simulink model "Modified_MIT_model_Ster_Adaptacyjne_am_2017b"  (R2021b)
settings: Solver=FixedStepAuto  StartTime=0.0  StopTime=100  FixedStep=0.001  RelTol=1e-3
values from neighbouring files (symbols this model uses):
  alpha = 1    [Modified_MIT_skrypt_Ster_Adaptacyjne_am.m]
  gamma = gamma_vec(i)    [Modified_MIT_skrypt_Ster_Adaptacyjne_am.m]    (also in skrypt_Ster_Adaptacyjne.m; skrypt_Ster_Adaptacyjne_2_rzedu.m; skrypt_Ster_Adaptacyjne_am.m)
  kd = 0.01    [Modified_MIT_skrypt_Ster_Adaptacyjne_am.m]
  ki = 1    [Modified_MIT_skrypt_Ster_Adaptacyjne_am.m]
  kp = 5    [Modified_MIT_skrypt_Ster_Adaptacyjne_am.m]
libraries: slpidlib x2
settings Model: Creator=marci  LastModifiedBy=marci
settings DebuggingCC: UnconnectedInputMsg=none  UnconnectedOutputMsg=none  UnconnectedLineMsg=none
settings RTWCC: DLArmComputeVersion=20.02.1

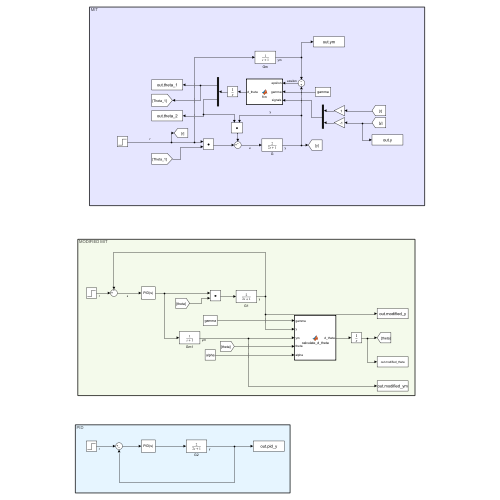
[thumbnail: Simulink's stored preview of the top-level diagram]
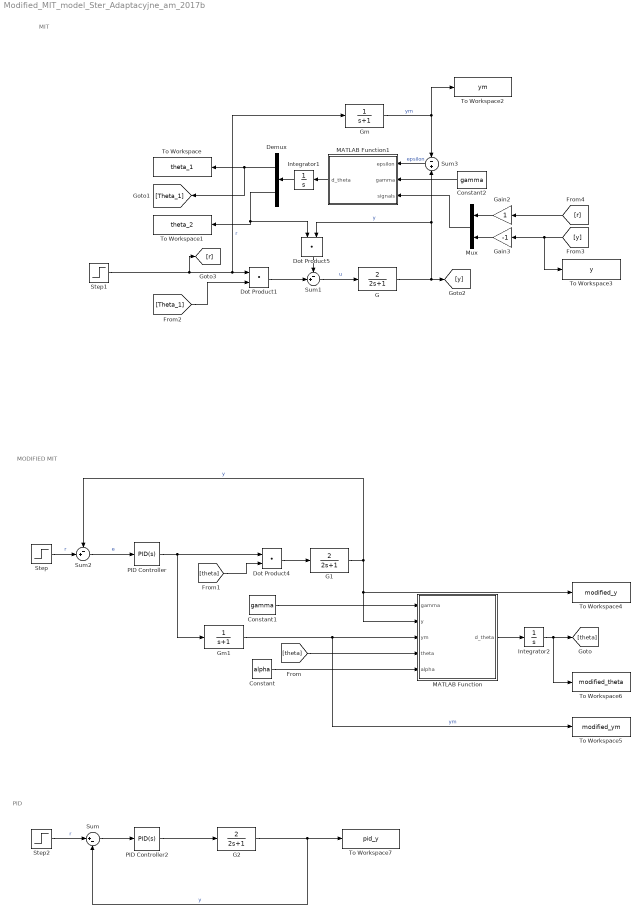
== system Modified_MIT_model_Ster_Adaptacyjne_am_2017b ==
  note: PID
  note: MODIFIED MIT
  note: MIT
  Constant : Constant  Value=alpha
  Constant1 : Constant  Value=gamma
  Constant2 : Constant  Value=gamma
  Demux : Demux  Outputs=2
  Dot Product1 : DotProduct  InputSameDT=on  OutDataTypeStr=Inherit: Inherit via internal rule
  Dot Product4 : DotProduct  InputSameDT=on  OutDataTypeStr=Inherit: Inherit via internal rule
  Dot Product5 : DotProduct  InputSameDT=on  OutDataTypeStr=Inherit: Inherit via internal rule
  G : TransferFcn  Numerator=[2]  Denominator=[2 1]
  G1 : TransferFcn  Numerator=[2]  Denominator=[2 1]
  G2 : TransferFcn  Numerator=[2]  Denominator=[2 1]
  Gain2 : Gain
  Gain3 : Gain  Gain=-1
  Gm : TransferFcn  Denominator=[1 1]
  Gm1 : TransferFcn  Denominator=[1 1]
  Integrator1 : Integrator
  Integrator2 : Integrator  InitialCondition=0.00001
  MATLAB Function : MATLAB Function  TreatAsAtomicUnit=on
  MATLAB Function1 : MATLAB Function  TreatAsAtomicUnit=on
  Mux : Mux  Inputs=2
  PID Controller : slpidlib/PID Controller  Controller=PID  Form=Parallel  TimeDomain=Continuous-time  UseExternalTs=off  SampleTime=-1  IntegratorMethod=Forward Euler  FilterMethod=Forward Euler  ControllerParametersSource=internal  P=kp  I=ki  D=kd  N=100  UseFilter=on  TunerSelectOption=Transfer Function Based (PID Tuner App)  InitialConditionSource=internal  InitialConditionForIntegrator=0  InitialConditionForFilter=0  DifferentiatorICPrevScaledInput=0  ExternalReset=none  TrackingMode=off  Kt=1  LimitOutput=off  SatLimitsSource=internal  UpperSaturationLimit=inf  LowerSaturationLimit=-inf  LinearizeAsGain=on  AntiWindupMode=none  Kb=1  POutMin=[]  POutMax=[]  IOutMin=[]  IOutMax=[]  DOutMin=[]  DOutMax=[]  NOutMin=[]  NOutMax=[]  SumOutMin=[]  SumOutMax=[]  SaturationOutMin=[]  SaturationOutMax=[]  PParamMin=[]  PParamMax=[]  IParamMin=[]  IParamMax=[]  DParamMin=[]  DParamMax=[]  NParamMin=[]  NParamMax=[]  KbParamMin=[]  KbParamMax=[]  KtParamMin=[]  KtParamMax=[]  KbOutMin=[]  KbOutMax=[]  KtOutMin=[]  KtOutMax=[]  IntegratorOutMin=[]  IntegratorOutMax=[]  FilterOutMin=[]  FilterOutMax=[]  SumI1OutMin=[]  SumI1OutMax=[]  SumI2OutMin=[]  SumI2OutMax=[]  SumI3OutMin=[]  SumI3OutMax=[]  SumI4OutMin=[]  SumI4OutMax=[]  SumDOutMin=[]  SumDOutMax=[]  DifferentiatorOutMin=[]  DifferentiatorOutMax=[]  FilterDiffOutCoefMin=[]  FilterDiffOutCoefMax=[]  ReciprocalOutMin=[]  ReciprocalOutMax=[]  SumDenOutMin=[]  SumDenOutMax=[]  SumNumOutMin=[]  SumNumOutMax=[]  DivideOutMin=[]  DivideOutMax=[]  UdiffTsProdOutMin=[]  UdiffTsProdOutMax=[]  NTsProdOutMin=[]  NTsProdOutMax=[]  UintegralTsProdOutMin=[]  UintegralTsProdOutMax=[]  UngainTsProdOutMin=[]  UngainTsProdOutMax=[]  IntegratorContinuousStateAttributes=''  IntegratorStateMustResolveToSignalObject=off  IntegratorRTWStateStorageClass=Auto  FilterContinuousStateAttributes=''  FilterStateMustResolveToSignalObject=off  FilterRTWStateStorageClass=Auto  ParallelPVariant=InternalParameters  IdealPVariant=Disabled  IVariant=InternalParameters  DVariant=InternalParameters  IntegratorVariant=Continuous  SatVariant=Disabled  AWVariant=Passthrough  PCopyVariant=Disabled  TRVariant=Disabled  FdbkBlocksVariant=Forward  IdealPFdbkVariant=Disabled  SatFdbkVariant=Disabled  DerivativeFilterVariant=ContFilter  NVariant=InternalParameters  NCopyVariant=Disabled  FilterICVariant=InternalICsFilter  IntegratorICVariant=InternalICs  ExternalResetVariant=Disabled  TRSumVariant=Passthrough  SumFdbkVariant=Disabled  SumVariant=Sum_PID  TsampFilterVariant=InternalTs  TsampNgainVariant=Passthrough  TsampIntegralVariant=Passthrough  ExternalSaturationOutDataTypeStr=Inherit: Same as second input
  PID Controller2 : slpidlib/PID Controller  Controller=PID  Form=Parallel  TimeDomain=Continuous-time  UseExternalTs=off  SampleTime=-1  IntegratorMethod=Forward Euler  FilterMethod=Forward Euler  ControllerParametersSource=internal  P=kp  I=ki  D=kd  N=100  UseFilter=on  TunerSelectOption=Transfer Function Based (PID Tuner App)  InitialConditionSource=internal  InitialConditionForIntegrator=0  InitialConditionForFilter=0  DifferentiatorICPrevScaledInput=0  ExternalReset=none  TrackingMode=off  Kt=1  LimitOutput=off  SatLimitsSource=internal  UpperSaturationLimit=inf  LowerSaturationLimit=-inf  LinearizeAsGain=on  AntiWindupMode=none  Kb=1  POutMin=[]  POutMax=[]  IOutMin=[]  IOutMax=[]  DOutMin=[]  DOutMax=[]  NOutMin=[]  NOutMax=[]  SumOutMin=[]  SumOutMax=[]  SaturationOutMin=[]  SaturationOutMax=[]  PParamMin=[]  PParamMax=[]  IParamMin=[]  IParamMax=[]  DParamMin=[]  DParamMax=[]  NParamMin=[]  NParamMax=[]  KbParamMin=[]  KbParamMax=[]  KtParamMin=[]  KtParamMax=[]  KbOutMin=[]  KbOutMax=[]  KtOutMin=[]  KtOutMax=[]  IntegratorOutMin=[]  IntegratorOutMax=[]  FilterOutMin=[]  FilterOutMax=[]  SumI1OutMin=[]  SumI1OutMax=[]  SumI2OutMin=[]  SumI2OutMax=[]  SumI3OutMin=[]  SumI3OutMax=[]  SumI4OutMin=[]  SumI4OutMax=[]  SumDOutMin=[]  SumDOutMax=[]  DifferentiatorOutMin=[]  DifferentiatorOutMax=[]  FilterDiffOutCoefMin=[]  FilterDiffOutCoefMax=[]  ReciprocalOutMin=[]  ReciprocalOutMax=[]  SumDenOutMin=[]  SumDenOutMax=[]  SumNumOutMin=[]  SumNumOutMax=[]  DivideOutMin=[]  DivideOutMax=[]  UdiffTsProdOutMin=[]  UdiffTsProdOutMax=[]  NTsProdOutMin=[]  NTsProdOutMax=[]  UintegralTsProdOutMin=[]  UintegralTsProdOutMax=[]  UngainTsProdOutMin=[]  UngainTsProdOutMax=[]  IntegratorContinuousStateAttributes=''  IntegratorStateMustResolveToSignalObject=off  IntegratorRTWStateStorageClass=Auto  FilterContinuousStateAttributes=''  FilterStateMustResolveToSignalObject=off  FilterRTWStateStorageClass=Auto  ParallelPVariant=InternalParameters  IdealPVariant=Disabled  IVariant=InternalParameters  DVariant=InternalParameters  IntegratorVariant=Continuous  SatVariant=Disabled  AWVariant=Passthrough  PCopyVariant=Disabled  TRVariant=Disabled  FdbkBlocksVariant=Forward  IdealPFdbkVariant=Disabled  SatFdbkVariant=Disabled  DerivativeFilterVariant=ContFilter  NVariant=InternalParameters  NCopyVariant=Disabled  FilterICVariant=InternalICsFilter  IntegratorICVariant=InternalICs  ExternalResetVariant=Disabled  TRSumVariant=Passthrough  SumFdbkVariant=Disabled  SumVariant=Sum_PID  TsampFilterVariant=InternalTs  TsampNgainVariant=Passthrough  TsampIntegralVariant=Passthrough  ExternalSaturationOutDataTypeStr=Inherit: Same as second input
  Step : Step  SampleTime=0
  Step1 : Step  SampleTime=0
  Step2 : Step  SampleTime=0
  Sum : Sum  Inputs=|+-
  Sum1 : Sum  Inputs=-+|
  Sum2 : Sum  Inputs=-+|
  Sum3 : Sum  Inputs=-+
  To Workspace : ToWorkspace  VariableName=theta_1  SaveFormat=Timeseries  SampleTime=-1
  To Workspace1 : ToWorkspace  VariableName=theta_2  SaveFormat=Timeseries  SampleTime=-1
  To Workspace2 : ToWorkspace  VariableName=ym  SaveFormat=Timeseries  SampleTime=-1
  To Workspace3 : ToWorkspace  VariableName=y  SaveFormat=Timeseries  SampleTime=-1
  To Workspace4 : ToWorkspace  VariableName=modified_y  SaveFormat=Timeseries  SampleTime=-1
  To Workspace5 : ToWorkspace  VariableName=modified_ym  SaveFormat=Timeseries  SampleTime=-1
  To Workspace6 : ToWorkspace  VariableName=modified_theta  SaveFormat=Timeseries  SampleTime=-1
  To Workspace7 : ToWorkspace  VariableName=pid_y  SaveFormat=Timeseries  SampleTime=-1
  wires:
  PID Controller/1 -> Gm1/1, Dot Product4/1
  Sum2/1 -> PID Controller/1  "e"
  Gm1/1 -> To Workspace5/1, MATLAB Function/3(ym)  "ym"
  Step/1 -> Sum2/2  "r"
  Dot Product4/1 -> G1/1
  G1/1 -> To Workspace4/1, MATLAB Function/2(y), Sum2/1  "y"
  MATLAB Function/1(d_theta) -> Integrator2/1
  Integrator2/1 -> To Workspace6/1, [theta]
  [theta] -> MATLAB Function/4(theta)
  Constant/1 -> MATLAB Function/5(alpha)
  Constant1/1 -> MATLAB Function/1(gamma)
  [theta] -> Dot Product4/2
  [y] -> To Workspace3/1, Gain3/1
  Gain3/1 -> Mux/2
  Gain2/1 -> Mux/1
  Demux/2 -> To Workspace1/1, Dot Product5/1
  G/1 -> [y], Dot Product5/2, Sum3/2  "y"
  [r] -> Gain2/1
  [Theta_1] -> Dot Product1/2
  Dot Product5/1 -> Sum1/1
  Gm/1 -> Sum3/1, To Workspace2/1  "ym"
  Dot Product1/1 -> Sum1/2
  MATLAB Function1/1(d_theta) -> Integrator1/1
  Step1/1 -> [r], Gm/1, Dot Product1/1  "r"
  Constant2/1 -> MATLAB Function1/2(gamma)
  Integrator1/1 -> Demux/1
  Mux/1 -> MATLAB Function1/3(signals)
  Sum1/1 -> G/1  "u"
  Sum3/1 -> MATLAB Function1/1(epsilon)  "epsilon"
  Demux/1 -> [Theta_1], To Workspace/1
  Step2/1 -> Sum/1  "r"
  Sum/1 -> PID Controller2/1
  PID Controller2/1 -> G2/1
  G2/1 -> To Workspace7/1, Sum/2  "y"

== matlab function Modified_MIT_model_Ster_Adaptacyjne_am_2017b/MATLAB Function1 ==
  data: epsilon input; d_theta output; gamma input; signals input
function d_theta = fcn(epsilon,gamma,signals)

d_theta = -gamma*epsilon*signals;

== matlab function Modified_MIT_model_Ster_Adaptacyjne_am_2017b/MATLAB Function ==
  data: gamma input; d_theta output; y input; ym input; theta input; alpha input
function d_theta = calculate_d_theta(gamma, y, ym, theta, alpha)

d_theta = -(gamma*(y-ym)*y/theta)/(alpha+(y/theta)^2);
